simulink model "quarter_car_model"  (R2026a)
settings: Solver=VariableStepAuto
undefined symbols (not defined in the file or in its folder): qc_params
settings Model: Creator=srp07  LastModifiedBy=srp07

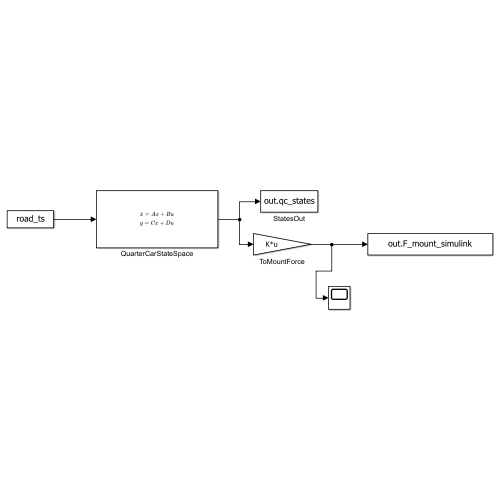
[thumbnail: Simulink's stored preview of the top-level diagram]
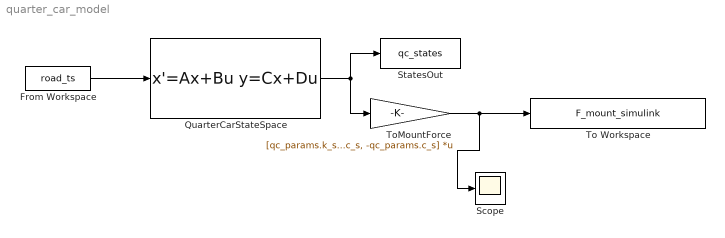
== system quarter_car_model ==
  From Workspace : FromWorkspace  VariableName=road_ts
  QuarterCarStateSpace : StateSpace  A=[0 0 1 0;0 0 0 1;-100 100 -7.14285714285714 7.14285714285714;777.777777777778 -6333.33333333333 55.5555555555556 -55.5555555555556]  B=[0;0;0;5555.55555555556]  C=[1 0 0 0;0 1 0 0;0 0 1 0;0 0 0 1]  D=[0;0;0;0]  InitialCondition=0
  Scope : Scope
      settings: ActiveDisplayYMinimum=-1  ActiveDisplayYMaximum=1
  StatesOut : ToWorkspace  VariableName=qc_states  SaveFormat=Timeseries  SampleTime=-1
  To Workspace : ToWorkspace  VariableName=F_mount_simulink  SaveFormat=Timeseries  SampleTime=-1
  ToMountForce : Gain  Gain=[qc_params.k_s, -qc_params.k_s, qc_params.c_s, -qc_params.c_s]  Multiplication=Matrix(K*u)
  wires:
  QuarterCarStateSpace/1 -> ToMountForce/1, StatesOut/1
  ToMountForce/1 -> Scope/1, To Workspace/1
  From Workspace/1 -> QuarterCarStateSpace/1
